simulink model "mpctmp_cl"  (R2023a)
settings: Solver=VariableStepAuto  StartTime=0.0  StopTime=100  RelTol=1e-3
values from neighbouring files (symbols this model uses):
  Fb0 = -(Cp0^2)/vp0/Gcd    (= 3.55555555556)    [mpctmp_init.m]
  Fbh0 = (ke*mlp0-dp0+vp0*Fb0/Cp0)/vp0    (= 6.82828282828)    [mpctmp_init.m]
  ke = -(dp0-((vp0/Cp0)^2)*Fb0*Gcv)/(mlp0-vp0*Glv)    (= 12.7272727273)    [mpctmp_init.m]
  ke2 = -((m2/Cs0)-M2-ds0)/mls0    (= 12.2245913291)    [mpctmp_init.m]
  kf = mlp0/(vp0*Fb0*Cp0*(1.2-0.3*gp0))    (= 0.20751953125)    [mpctmp_init.m]
  kf2 = mls0/(m2*Cs0*(1.2-0.3*gs0))    (= 0.170918367347)    [mpctmp_init.m]
  m2 = vp0*Fb0    (= 106.666666667)    [mpctmp_init.m]
  M2 = vp0*Fbh0+dp0-ke*mlp0    (= 266.666666667)    [mpctmp_init.m]
libraries: cstblocks x9, simulink x4, mpclib x1
settings Model: Creator=The MathWorks, Inc.  LastModifiedBy=The MathWorks, Inc.
settings SolverCC: MaxZcPerStep=1
settings DebuggingCC: UnconnectedInputMsg=warning  UnconnectedOutputMsg=warning  UnconnectedLineMsg=warning
settings ModelReferenceCC: EnableRefExpFcnMdlSchedulingChecks=on
settings RTWCC: DLArmComputeVersion=19.05

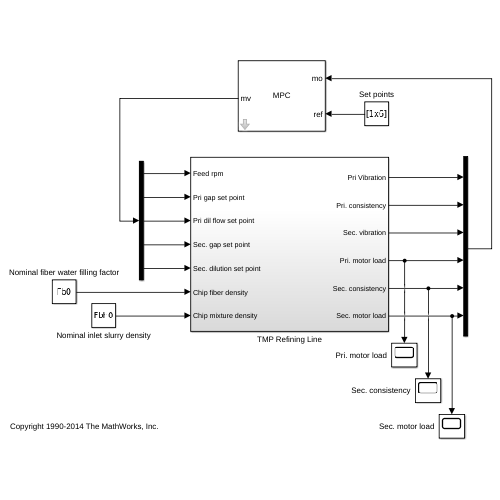
[thumbnail: Simulink's stored preview of the top-level diagram]
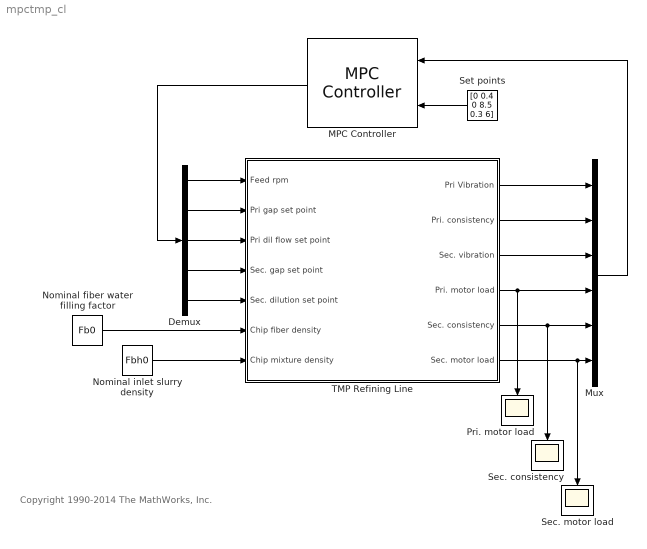
== system mpctmp_cl ==
  note: Copyright 1990-2014 The MathWorks, Inc.
  Demux : Demux  Outputs=5
  MPC Controller : mpclib/MPC Controller  mpcobj=mpcobj  x0=[]  is_multiple=0  enable_value=0  return_u0=off  updateMPCinCallerWorkspace=on  md_inport=off  mv_inport=off  uref_inport=off  return_cost=off  return_mvseq=off  return_qpstatus=off  return_xseq=off  return_state=off  return_ovseq=off  state_inport=off  umin_inport=off  umax_inport=off  ymin_inport=off  ymax_inport=off  cc_inport=off  ywt_inport=off  uwt_inport=off  duwt_inport=off  rhoeps_inport=off  pm_inport=off  MaximumP=10  HorizonChoice=FixedHorizon  n_ts=0.5  n_p=20  n_mv=5  n_md=0  n_ud=0  n_mo=6  n_uo=0  BlockDataType=double  SampleTimeInherited=off  switch_inport=off
  Mux : Mux  Inputs=6
  Nominal fiber water filling factor : Constant  Value=Fb0
  Nominal inlet slurry density : Constant  Value=Fbh0
  Pri. motor load : Scope
  Sec. consistency : Scope
  Sec. motor load : Scope
  Set points : Constant  Value=[0 0.4 0 8.5 0.3 6]
  TMP Refining Line : Subsystem
  wires:
  Nominal inlet slurry density/1 -> TMP Refining Line/7(Chip mixture density)
  MPC Controller/1 -> Demux/1
  Nominal fiber water filling factor/1 -> TMP Refining Line/6(Chip fiber density)
  Demux/2 -> TMP Refining Line/2(Pri gap set point)
  Set points/1 -> MPC Controller/2
  Mux/1 -> MPC Controller/1
  TMP Refining Line/6(Sec. motor load) -> Mux/6, Sec. motor load/1
  TMP Refining Line/5(Sec. consistency) -> Sec. consistency/1, Mux/5
  TMP Refining Line/4(Pri. motor load) -> Pri. motor load/1, Mux/4
  TMP Refining Line/3(Sec. vibration) -> Mux/3
  TMP Refining Line/2(Pri. consistency) -> Mux/2
  TMP Refining Line/1(Pri Vibration) -> Mux/1
  Demux/5 -> TMP Refining Line/5(Sec. dilution set point)
  Demux/4 -> TMP Refining Line/4(Sec. gap set point)
  Demux/3 -> TMP Refining Line/3(Pri dil flow set point)
  Demux/1 -> TMP Refining Line/1(Feed rpm)

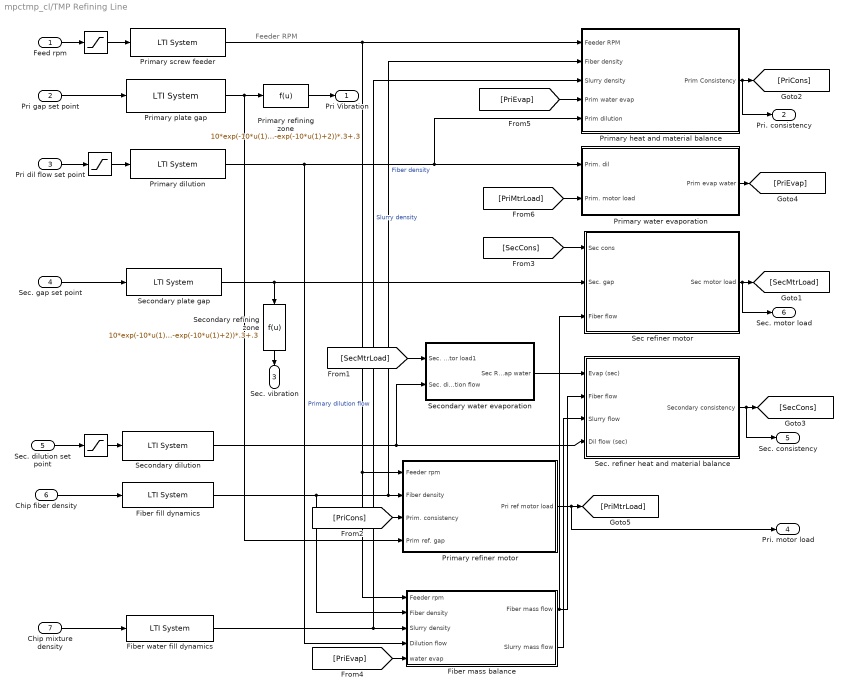
== system mpctmp_cl/TMP Refining Line ==
  note: Feeder RPM
  Feed rpm : Inport
  Pri gap set point : Inport  Port=2
  Pri dil flow set point : Inport  Port=3
  Sec. gap set point : Inport  Port=4
  Sec. dilution set point : Inport  Port=5
  Chip fiber density : Inport  Port=6
  Chip mixture density : Inport  Port=7
  "  " : Saturate  UpperLimit=35  LowerLimit=25  SampleTime=0.5
  "    " : Saturate  UpperLimit=200  LowerLimit=90  SampleTime=0.5
  "       " : Saturate  UpperLimit=200  LowerLimit=90  SampleTime=0.5
  Fiber fill dynamics : cstblocks/LTI System  sys=FiberFill  IC=Fb0
  Fiber mass balance : Subsystem
  Fiber water fill dynamics : cstblocks/LTI System  sys=FiberWaterFill  IC=Fbh0
  Primary dilution : cstblocks/LTI System  sys=DilFlowPrimary  IC=dp0
  Primary heat and material balance : Subsystem
  Primary plate gap : cstblocks/LTI System  sys=PlateGapPrimary  IC=gp0
  Primary refiner motor : Subsystem
  Primary refining zone : Fcn  Expr=10*exp(-10*u(1)+2)*(1.26-0.3*u(1))-(1-exp(-10*u(1)+2))*.3+.3
  Primary screw feeder : cstblocks/LTI System  sys=ChipFeeder  IC=vp0
  Primary water evaporation : Subsystem
  Sec refiner motor : Subsystem
  Sec. refiner heat and material balance : Subsystem
  "Secondary dilution " : cstblocks/LTI System  sys=DilFlowSecondary  IC=gs0
  Secondary plate gap : cstblocks/LTI System  sys=PlateGapSecondary  IC=gs0
  Secondary refining zone : Fcn  Expr=10*exp(-10*u(1)+2)*(1.26-0.3*u(1))-(1-exp(-10*u(1)+2))*.3+.3  SampleTime=0.5
  Secondary water evaporation : Subsystem
  Pri Vibration : Outport
  Pri. consistency : Outport  Port=2
  Sec. vibration : Outport  Port=3
  Pri. motor load : Outport  Port=4
  Sec. consistency : Outport  Port=5
  Sec. motor load : Outport  Port=6
  wires:
  Chip mixture density/1 -> Fiber water fill dynamics/1
  Chip fiber density/1 -> Fiber fill dynamics/1
  [PriEvap] -> Fiber mass balance/5(water evap)
  Secondary refining zone/1 -> Sec. vibration/1
  Sec. gap set point/1 -> Secondary plate gap/1
  Pri dil flow set point/1 -> "    "/1
  Pri gap set point/1 -> Primary plate gap/1
  Feed rpm/1 -> "  "/1
  [SecMtrLoad] -> Secondary water evaporation/1(Sec. motor load1)
  [PriMtrLoad] -> Primary water evaporation/2(Prim. motor load)
  Primary refiner motor/1(Pri ref motor load) -> Pri. motor load/1, [PriMtrLoad]
  [PriEvap] -> Primary heat and material balance/4(Prim water evap)
  Primary water evaporation/1(Prim evap water) -> [PriEvap]
  [SecCons] -> Sec refiner motor/1(Sec cons)
  Sec. refiner heat and material balance/1(Secondary consistency) -> Sec. consistency/1, [SecCons]
  [PriCons] -> Primary refiner motor/3(Prim. consistency)
  Primary heat and material balance/1(Prim Consistency) -> Pri. consistency/1, [PriCons]
  Sec refiner motor/1(Sec motor load) -> Sec. motor load/1, [SecMtrLoad]
  Primary refining zone/1 -> Pri Vibration/1
  Secondary water evaporation/1(Sec Ref. evap water) -> Sec. refiner heat and material balance/1(Evap (sec))
  Fiber mass balance/2(Slurry mass flow) -> Sec. refiner heat and material balance/3(Slurry flow)
  Fiber mass balance/1(Fiber mass flow) -> Sec refiner motor/3(Fiber flow), Sec. refiner heat and material balance/2(Fiber flow)
  Primary screw feeder/1 -> Primary refiner motor/1(Feeder rpm), Fiber mass balance/1(Feeder rpm), Primary heat and material balance/1(Feeder RPM)
  Primary dilution/1 -> Fiber mass balance/4(Dilution flow), Primary heat and material balance/5(Prim dilution), Primary water evaporation/1(Prim. dil)  "Primary dilution flow"
  Fiber fill dynamics/1 -> Primary refiner motor/2(Fiber density), Primary heat and material balance/2(Fiber density), Fiber mass balance/2(Fiber density)  "Fiber density"
  Fiber water fill dynamics/1 -> Fiber mass balance/3(Slurry density), Primary heat and material balance/3(Slurry density)  "Slurry density"
  Sec. dilution set point/1 -> "       "/1
  "Secondary dilution "/1 -> Secondary water evaporation/2(Sec. dilution flow), Sec. refiner heat and material balance/4(Dil flow (sec))
  "       "/1 -> "Secondary dilution "/1
  "    "/1 -> Primary dilution/1
  Secondary plate gap/1 -> Sec refiner motor/2(Sec. gap), Secondary refining zone/1
  Primary plate gap/1 -> Primary refiner motor/4(Prim ref. gap), Primary refining zone/1
  "  "/1 -> Primary screw feeder/1

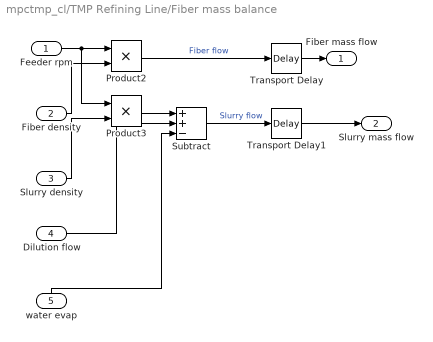
== system mpctmp_cl/TMP Refining Line/Fiber mass balance ==
  Feeder rpm : Inport
  Fiber density : Inport  Port=2
  Slurry density : Inport  Port=3
  Dilution flow : Inport  Port=4
  water evap : Inport  Port=5
  Product2 : Product  RndMeth=Zero
  Product3 : Product  RndMeth=Zero
  Subtract : Sum  Inputs=++-
  Transport Delay : TransportDelay  DelayTime=2  InitialOutput=m2
  Transport Delay1 : TransportDelay  DelayTime=2  InitialOutput=M2
  Fiber mass flow : Outport
  Slurry mass flow : Outport  Port=2
  wires:
  Transport Delay1/1 -> Slurry mass flow/1
  Transport Delay/1 -> Fiber mass flow/1
  water evap/1 -> Subtract/3
  Dilution flow/1 -> Subtract/2
  Slurry density/1 -> Product3/2
  Fiber density/1 -> Product2/2
  Feeder rpm/1 -> Product3/1, Product2/1
  Subtract/1 -> Transport Delay1/1  "Slurry flow"
  Product3/1 -> Subtract/1
  Product2/1 -> Transport Delay/1  "Fiber flow"

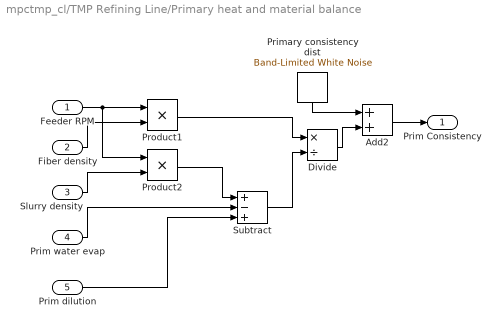
== system mpctmp_cl/TMP Refining Line/Primary heat and material balance ==
  Feeder RPM : Inport
  Fiber density : Inport  Port=2
  Slurry density : Inport  Port=3
  Prim water evap : Inport  Port=4
  Prim dilution : Inport  Port=5
  Add2 : Sum
  Divide : Product  Inputs=*/  SampleTime=.5
  Primary consistency dist : simulink/Sources/Band-Limited White Noise  Cov=0.00001  Ts=0.5  seed=[23341]
  Product1 : Product  RndMeth=Zero
  Product2 : Product  RndMeth=Zero
  Subtract : Sum  Inputs=+-+
  Prim Consistency : Outport
  wires:
  Prim water evap/1 -> Subtract/2
  Slurry density/1 -> Product2/2
  Fiber density/1 -> Product1/2
  Add2/1 -> Prim Consistency/1
  Prim dilution/1 -> Subtract/3
  Feeder RPM/1 -> Product2/1, Product1/1
  Primary consistency dist/1 -> Add2/1
  Divide/1 -> Add2/2
  Product1/1 -> Divide/1
  Subtract/1 -> Divide/2
  Product2/1 -> Subtract/1

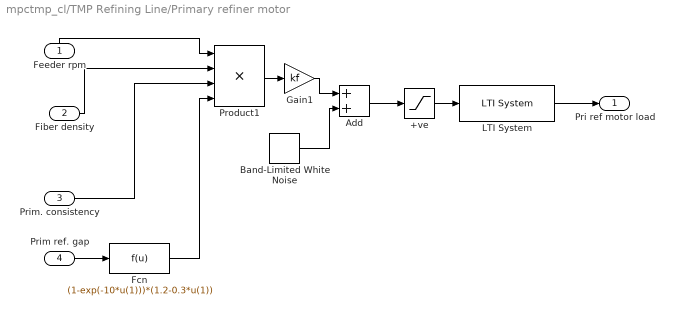
== system mpctmp_cl/TMP Refining Line/Primary refiner motor ==
  Feeder rpm : Inport
  Fiber density : Inport  Port=2
  Prim. consistency : Inport  Port=3
  Prim ref. gap : Inport  Port=4
  +ve : Saturate  UpperLimit=inf  LowerLimit=0  SampleTime=0.5
  Add : Sum
  Band-Limited White Noise : simulink/Sources/Band-Limited White Noise  Cov=0.0001  Ts=0.5  seed=[23341]
  Fcn : Fcn  Expr=(1-exp(-10*u(1)))*(1.2-0.3*u(1))
  Gain1 : Gain  Gain=kf
  LTI System : cstblocks/LTI System  sys=UnitDelay  IC=mlp0
  Product1 : Product  Inputs=4  RndMeth=Zero
  Pri ref motor load : Outport
  wires:
  LTI System/1 -> Pri ref motor load/1
  +ve/1 -> LTI System/1
  Prim. consistency/1 -> Product1/3
  Prim ref. gap/1 -> Fcn/1
  Fiber density/1 -> Product1/2
  Feeder rpm/1 -> Product1/1
  Band-Limited White Noise/1 -> Add/2
  Add/1 -> +ve/1
  Gain1/1 -> Add/1
  Fcn/1 -> Product1/4
  Product1/1 -> Gain1/1

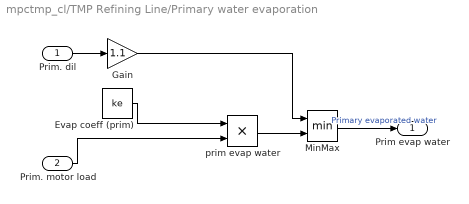
== system mpctmp_cl/TMP Refining Line/Primary water evaporation ==
  Prim. dil : Inport
  Prim. motor load : Inport  Port=2
  Evap coeff (prim) : Constant  Value=ke
  Gain : Gain  Gain=1.1
  MinMax : MinMax  Inputs=2
  prim evap water : Product  RndMeth=Zero
  Prim evap water : Outport
  wires:
  Prim. motor load/1 -> prim evap water/2
  MinMax/1 -> Prim evap water/1  "Primary evaporated water"
  Prim. dil/1 -> Gain/1
  Gain/1 -> MinMax/1
  prim evap water/1 -> MinMax/2
  Evap coeff (prim)/1 -> prim evap water/1

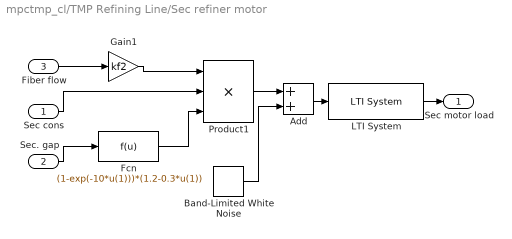
== system mpctmp_cl/TMP Refining Line/Sec refiner motor ==
  Sec cons : Inport
  Sec. gap : Inport  Port=2
  Fiber flow : Inport  Port=3
  Add : Sum
  Band-Limited White Noise : simulink/Sources/Band-Limited White Noise  Cov=0.0001  Ts=0.5  seed=[23341]
  Fcn : Fcn  Expr=(1-exp(-10*u(1)))*(1.2-0.3*u(1))
  Gain1 : Gain  Gain=kf2
  LTI System : cstblocks/LTI System  sys=UnitDelay  IC=mls0
  Product1 : Product  Inputs=3  RndMeth=Zero
  Sec motor load : Outport
  wires:
  LTI System/1 -> Sec motor load/1
  Add/1 -> LTI System/1
  Sec cons/1 -> Product1/2
  Sec. gap/1 -> Fcn/1
  Fiber flow/1 -> Gain1/1
  Band-Limited White Noise/1 -> Add/2
  Product1/1 -> Add/1
  Fcn/1 -> Product1/3
  Gain1/1 -> Product1/1

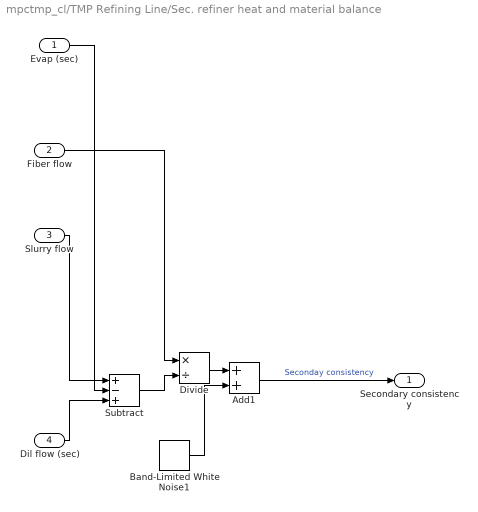
== system mpctmp_cl/TMP Refining Line/Sec. refiner heat and material balance ==
  Evap (sec) : Inport
  Fiber flow : Inport  Port=2
  Slurry flow : Inport  Port=3
  Dil flow (sec) : Inport  Port=4
  Add1 : Sum
  Band-Limited White Noise1 : simulink/Sources/Band-Limited White Noise  Cov=0.00001  Ts=0.5  seed=[23341]
  Divide : Product  Inputs=*/  SampleTime=.5
  Subtract : Sum  Inputs=+-+
  Secondary consistency : Outport
  wires:
  Slurry flow/1 -> Subtract/1
  Add1/1 -> Secondary consistency/1  "Seconday consistency"
  Dil flow (sec)/1 -> Subtract/3
  Fiber flow/1 -> Divide/1
  Band-Limited White Noise1/1 -> Add1/2
  Divide/1 -> Add1/1
  Subtract/1 -> Divide/2
  Evap (sec)/1 -> Subtract/2

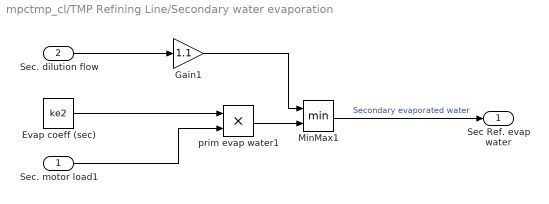
== system mpctmp_cl/TMP Refining Line/Secondary water evaporation ==
  Sec. motor load1 : Inport
  Sec. dilution flow : Inport  Port=2
  Evap coeff (sec) : Constant  Value=ke2
  Gain1 : Gain  Gain=1.1
  MinMax1 : MinMax  Inputs=2
  prim evap water1 : Product  RndMeth=Zero
  Sec Ref. evap water : Outport
  wires:
  MinMax1/1 -> Sec Ref. evap water/1  "Secondary evaporated water"
  Gain1/1 -> MinMax1/1
  Sec. motor load1/1 -> prim evap water1/2
  Sec. dilution flow/1 -> Gain1/1
  prim evap water1/1 -> MinMax1/2
  Evap coeff (sec)/1 -> prim evap water1/1
